simulink model "ElectricVehicleNMPC"  (R2022b)
settings: Solver=VariableStepAuto  StartTime=0  StopTime=600+N*Ts  RelTol=1e-3
model workspace (MAT data in the model file):
  AccessaryLoad : Simulink.Parameter (value not decoded)
  BrakeRegenFraction : Simulink.Parameter (value not decoded)
  Crr : Simulink.Parameter (value not decoded)
  DrivelineModelG : Simulink.Parameter (value not decoded)
  DrivelineModelSpinLoss : Simulink.Parameter (value not decoded)
  EnergyCapacity : Simulink.Parameter (value not decoded)
  MassVehInertia : Simulink.Parameter (value not decoded)
  MaxPowerOutput : Simulink.Parameter (value not decoded)
  MaxTorqueOutput : Simulink.Parameter (value not decoded)
  MaximumBreakForce : Simulink.Parameter (value not decoded)
  MotorModelC : Simulink.Parameter (value not decoded)
  MotorModelKc : Simulink.Parameter (value not decoded)
  MotorModelKi : Simulink.Parameter (value not decoded)
  MotorModelKw : Simulink.Parameter (value not decoded)
  N : Simulink.Parameter (value not decoded)
  Q : Simulink.Parameter (value not decoded)
  Rint : Simulink.Parameter (value not decoded)
  Ts : Simulink.Parameter (value not decoded)
  Voc : Simulink.Parameter (value not decoded)
  gravity : Simulink.Parameter (value not decoded)
  massVeh : Simulink.Parameter (value not decoded)
  theta : Simulink.Parameter (value not decoded)
  wheelRadius : Simulink.Parameter (value not decoded)
values from neighbouring files (symbols this model uses):
  AccessaryLoad = 600    [NMPC_EV.m]
  BrakeRegenFraction = 0.55    [NMPC_EV.m]
  Crr = 0.01    [NMPC_EV.m]
  DrivelineModelG = 3.55    [NMPC_EV.m]
  DrivelineModelSpinLoss = 6    [NMPC_EV.m]
  EnergyCapacity = 12.6    [NMPC_EV.m]
  gravity = 9.81    [NMPC_EV.m]
  m = 2    [NMPC_EV.m]
  massVeh = 2300    [NMPC_EV.m]
  MassVehInertia = 2392    [NMPC_EV.m]
  MaximumBreakForce = 10000    [NMPC_EV.m]
  MaxPowerOutput = 1e5    (= 100000)    [NMPC_EV.m]
  MaxTorqueOutput = 500    [NMPC_EV.m]
  MotorModelC = 628.2974    [NMPC_EV.m]
  MotorModelKc = 0.045237    [NMPC_EV.m]
  MotorModelKi = 0.0167    [NMPC_EV.m]
  MotorModelKw = 5.06640055940796E-5    (= 5.06640055941e-05)    [NMPC_EV.m]
  N = 5    [NMPC_EV.m]
  Q = 3000    [NMPC_EV.m]
  Rint = 0.1    [NMPC_EV.m]
  Ts = 0.01    [NMPC_EV.m]
  Voc = 340    [NMPC_EV.m]
  wheelRadius = 0.34    [NMPC_EV.m]
symbols that are objects in the model workspace (value not decoded): theta
libraries: simulink x12, autolibshared x2
(part 2 of 2)

== matlab function ElectricVehicleNMPC/NMPC1/MATLAB Function ==
  settings: updateMethod=DISCRETE
  data: Vahead input; Vref input; Pt output; FB output; VehicleV input; soc input; N data_store_memory; BrakeRegenFraction data_store_memory; Crr data_store_memory; DrivelineModelG data_store_memory; DrivelineModelSpinLoss data_store_memory; EnergyCapacity data_store_memory; MassVehInertia data_store_memory; MotorModelC data_store_memory; MotorModelKc data_store_memory; MotorModelKi data_store_memory; MotorModelKw data_store_memory; Rint data_store_memory; Voc data_store_memory; massVeh data_store_memory; wheelRadius data_store_memory; AccessaryLoad data_store_memory; Ts data_store_memory; gravity data_store_memory; Q data_store_memory; MaxTorqueOutput data_store_memory; n data_store_memory; m data_store_memory; vr data_store_memory; v data_store_memory; SOC data_store_memory; SOCr data_store_memory; Ptr data_store_memory; FBr data_store_memory; MaxPowerOutput data_store_memory; Vpre data_store_memory
function [Pt,FB] = fcn(Vahead,Vref,VehicleV,soc)
% u1 = Pt Positive Torque
% u2 = FB Total BrakeForce


global AccessaryLoad BrakeRegenFraction Crr DrivelineModelG DrivelineModelSpinLoss EnergyCapacity MassVehInertia MotorModelC
global MotorModelKc MotorModelKi MotorModelKw Rint Voc massVeh wheelRadius MaxTorqueOutput MaxPowerOutput
global N Ts Q
global n m vr v Ptr FBr SOC SOCr Vpre

persistent Vtrajectory zek G_rw u1 u2
persistent xmin xmax umin Fx Fu R Qx QX RU FX FU F H
if isempty(u1)
    G_rw = DrivelineModelG/wheelRadius;
    Vtrajectory = zeros(N+1,1); % +1 to include current reference
    zek = [zeros(n*(N+1),1);zeros(m*N,1)];

    xmin = [-1e5;5]; xmax = [1e5;100]; 
    umin = [0;-1e4];
    Fx = [0 0;0 1;0 0;0 -1]; % No constraints on velcity
    Fu = [eye(m);-eye(m)]; R = eye(m);
    Qx = [Q 0;0 1];
    QX = zeros(n*(N+1),n*(N+1));
    RU = zeros(m*N,m*N);
    FX = zeros(2*n*(N+1),n*(N+1));
    FU = zeros(2*m*N,m*N);
    for i = 1:N
        QX((i-1)*n+1:i*n,(i-1)*n+1:i*n) = Qx;
        RU((i-1)*m+1:i*m,(i-1)*m+1:i*m) = R;

        FX((i-1)*2*n+1:i*2*n,(i-1)*n+1:i*n) = Fx;
        FU((i-1)*2*m+1:i*2*m,(i-1)*m+1:i*m) = Fu;
    end
    QX(N*n+1:end,N*n+1:end) = Qx;
    FX(N*2*n+1:end,N*n+1:end) = Fx;
    F = blkdiag(FX,FU);
    H = blkdiag(QX,RU.*0); 

    SOCr=100;
    u1=0;u2=0;
end

Vtrajectory(1:end-1,1) = Vtrajectory(2:end,1);
Vtrajectory(end,1) = Vahead;
% Vpre = Vtrajectory; % from persistent variable to global variable
Vpre = zeros(11,1);
for i =1:N+1
    Vpre(i)=Vtrajectory(i,1);
end
vr = Vref; v = VehicleV; SOC = soc; 

MotorSpeed = max(G_rw*abs(v),1e-5); % MotorSpeed must be positive
umax = [min(MaxTorqueOutput,MaxPowerOutput/MotorSpeed);0];

Gxe = zeros(2*n*(N+1),1);
Gue = zeros(2*m*N,1);
Ptr=zeros(11,1);FBr=zeros(11,1);
Pt=u1;FB=u2;
for i = 1:N
    xr = [Vtrajectory(i,1);SOCr]; %future references
    [Pt,FB] = desiredControl(xr(1),Vtrajectory(i+1),Pt,FB); % Find equilibrium control using fd
    Ptr(i,1)=Pt;FBr(i,1)=FB;

    gxe = [xmax;-xmin] - Fx*xr;
    gue = [umax;-umin] - Fu*[Pt;FB];

    Gxe((i-1)*2*n+1:i*2*n,1) = gxe;
    Gue((i-1)*2*m+1:i*2*m,1) = gue;
end
xr = [Vtrajectory(end,1);SOCr]; %future references
[Ptr(end,1),FBr(end,1)] = desiredControl(xr(1),xr(1),Pt,FB);
gxe = [xmax;-xmin] - Fx*xr;
Gxe(N*2*n+1:end,1) = gxe;

% Simulation with NMPC
ObjFunc = @(ze) (ze'*H*ze);
G = [Gxe;Gue];
nonlcon = @NonlinearConstraints;
options = optimoptions('fmincon','Algorithm','sqp');
zek = fmincon(ObjFunc,zek,F,G,[],[],[],[],nonlcon,options);
u = zek(n*(N+1)+1:n*(N+1)+m,1) + [Ptr(1,1);FBr(1,1)];
% if(abs(vr)==abs(v))
%     u1=0;u2=0;
% elseif(vr>v)
%     u1=u(1);
%     u2=0;
% else
%     u1=0;
%     u2=u(2);
% end
if(abs(vr)==abs(v)&&abs(v)==0)
    u1=0;u2=0;
else
    u1=u(1);u2=u(2);
end
Pt = u1;
FB = u2;
end


%%%%%%%%%%%%%%%%%%%%%%%%%%%%%%%%%%%%%%%%%%%%%%%%%%%%%%%%%%%%%%%%%%%%%%%%%%%
%%%%%%%%%%%%%%%%%%%%%%%%%%%%%%%%%%%%%%%%%%%%%%%%%%%%%%%%%%%%%%%%%%%%%%%%%%%
function [Ptr, FBr] = desiredControl(vr,vr1,Pt,FB)
global massVeh gravity Crr DrivelineModelSpinLoss DrivelineModelG wheelRadius MassVehInertia
global BrakeRegenFraction AccessaryLoad  MotorModelKc MotorModelKw MotorModelKi MotorModelC Ts

G_rw = DrivelineModelG/wheelRadius;
C1 = 0.5*vr^2 + massVeh*gravity*Crr + DrivelineModelSpinLoss*G_rw;
C2 = AccessaryLoad + MotorModelKw*(G_rw*vr)^3 + MotorModelKi*G_rw*vr + MotorModelC;
root = roots([MotorModelKc,G_rw*vr,C2]);
if(isreal(root))
    TM_r = max(root);
    u2r = C1 - TM_r*G_rw + (vr1-vr)*MassVehInertia/Ts;
    u1r = TM_r + BrakeRegenFraction/G_rw*u2r;

%     Ptr = max(0,u1r);
%     FBr = min(0,u2r);
    Ptr = u1r;
    FBr = u2r;
else
    Ptr = Pt;
    FBr = FB;
end

end

function [c,ceq] = NonlinearConstraints(z)
global v SOC SOCr Ptr FBr Vpre
global N n m
c=[];
shift = n*(N+1);
c1 = zeros(n*N,1);
for i=1:N
    vz = z(n*(i-1)+1,1);
    socz = z(i*n,1);
    Ptz = z(shift+m*(i-1)+1,1);
    FBz = z(shift+i*m,1);
    Pt_r = Ptr(i);FB_r=FBr(i);v_r=Vpre(i,1);
    [v1,soc1] = fd2(vz+v_r,socz+SOCr,Ptz+Pt_r,FBz+FB_r);
    c1(n*(i-1)+1) = z(i*n+1,1)+v_r - v1;
    c1(n*i) = z((i+1)*n,1)+SOCr - soc1;
end
ceq = [z(1)+Vpre(1,1)-v;z(2)+SOCr-SOC;c1];
end

function [v_prime,soc_prime] = fd2(v,SOC,PositiveTorque,FB)
global Ts
[dv1,dsoc1] = fc(v,PositiveTorque,FB);
v_prime = v + Ts*dv1;
soc_prime = SOC + Ts*dsoc1;
end

function [dv,dsoc] = fc(v,PositiveTorque,FB)
global MassVehInertia massVeh gravity Crr DrivelineModelSpinLoss DrivelineModelG
global wheelRadius BrakeRegenFraction Voc EnergyCapacity MaxTorqueOutput MaxPowerOutput

G_wr = DrivelineModelG/wheelRadius;
MotorSpeed = max(G_wr*abs(v),1e-5);
if(abs(v)<2.2352) % less than 2.2352 m/s = 5mph
    RegenTorque = 0;
else
    RegenTorque = BrakeRegenFraction*FB/G_wr; % Negative
    RegenTorque = max(RegenTorque,-0.5*min(MaxTorqueOutput,MaxPowerOutput/MotorSpeed));
end
BrakeForce = max((1-BrakeRegenFraction)*FB,-1e4);
MotorTorque = PositiveTorque + RegenTorque;
if(abs(v)~=0)
    TractiveForce = (MotorTorque - DrivelineModelSpinLoss)*G_wr  + BrakeForce;
    RollingResistence = massVeh*gravity*Crr;
else
    TractiveForce = MotorTorque*G_wr  + BrakeForce;
    RollingResistence = 0;
end
dv = (TractiveForce - 0.5*v^2 -RollingResistence)/MassVehInertia;
P = MotorPower(MotorTorque,MotorSpeed);
I = Current(P);
dsoc = -Voc*I/(EnergyCapacity*1000*3600)*100;% in %
end

function P = MotorPower(MotorTorque,MotorSpeed)
global AccessaryLoad  MotorModelKc MotorModelKw MotorModelKi MotorModelC 
if(MotorSpeed>1e-3)
    Powerloss = MotorModelKc*MotorTorque^2 +... 
         MotorModelKw*(MotorSpeed)^3 + MotorModelKi*MotorSpeed + MotorModelC;
else
    Powerloss =  0;
end
P = Powerloss + MotorSpeed*MotorTorque + AccessaryLoad;
end

function I = Current(P)
global Voc Rint
dummy = Voc^2 - 4*Rint*P;
I = (Voc - sqrt(dummy))/(2*Rint);
end

== matlab function ElectricVehicleNMPC/NMPC/MATLAB Function ==
  settings: updateMethod=DISCRETE
  data: Vahead input; Vref input; Pt output; FB output; VehicleV input; soc input; N data_store_memory; BrakeRegenFraction data_store_memory; Crr data_store_memory; DrivelineModelG data_store_memory; DrivelineModelSpinLoss data_store_memory; EnergyCapacity data_store_memory; MassVehInertia data_store_memory; MotorModelC data_store_memory; MotorModelKc data_store_memory; MotorModelKi data_store_memory; MotorModelKw data_store_memory; Rint data_store_memory; Voc data_store_memory; massVeh data_store_memory; wheelRadius data_store_memory; AccessaryLoad data_store_memory; Ts data_store_memory; gravity data_store_memory; Q data_store_memory; MaxTorqueOutput data_store_memory; n data_store_memory; m data_store_memory; vr data_store_memory; v data_store_memory; SOC data_store_memory; SOCr data_store_memory; Ptr data_store_memory; FBr data_store_memory; MaxPowerOutput data_store_memory; Vpre data_store_memory
function [Pt,FB] = fcn(Vahead,Vref,VehicleV,soc)
% u1 = Pt Positive Torque
% u2 = FB Total BrakeForce


global AccessaryLoad BrakeRegenFraction Crr DrivelineModelG DrivelineModelSpinLoss EnergyCapacity MassVehInertia MotorModelC
global MotorModelKc MotorModelKi MotorModelKw Rint Voc massVeh wheelRadius MaxTorqueOutput MaxPowerOutput
global N Ts Q
global n m vr v Ptr FBr SOC SOCr Vpre

persistent Vtrajectory zek G_rw u1 u2
persistent xmin xmax umin Fx Fu R Qx QX RU FX FU F H
if isempty(u1)
    G_rw = DrivelineModelG/wheelRadius;
    Vtrajectory = zeros(N+1,1); % +1 to include current reference
    zek = [zeros(n*(N+1),1);zeros(m*N,1)];

    xmin = [-1e5;5]; xmax = [1e5;100]; 
    umin = [0;-1e4];
    Fx = [0 0;0 1;0 0;0 -1]; % No constraints on velcity
    Fu = [eye(m);-eye(m)]; R = eye(m);
    Qx = [Q 0;0 1];
    QX = zeros(n*(N+1),n*(N+1));
    RU = zeros(m*N,m*N);
    FX = zeros(2*n*(N+1),n*(N+1));
    FU = zeros(2*m*N,m*N);
    for i = 1:N
        QX((i-1)*n+1:i*n,(i-1)*n+1:i*n) = Qx;
        RU((i-1)*m+1:i*m,(i-1)*m+1:i*m) = R;

        FX((i-1)*2*n+1:i*2*n,(i-1)*n+1:i*n) = Fx;
        FU((i-1)*2*m+1:i*2*m,(i-1)*m+1:i*m) = Fu;
    end
    QX(N*n+1:end,N*n+1:end) = Qx;
    FX(N*2*n+1:end,N*n+1:end) = Fx;
    F = blkdiag(FX,FU);
    H = blkdiag(QX,RU.*0); 

    SOCr=100;
    u1=0;u2=0;
end

Vtrajectory(1:end-1,1) = Vtrajectory(2:end,1);
Vtrajectory(end,1) = Vahead;
% Vpre = Vtrajectory; % from persistent variable to global variable
Vpre = zeros(11,1);
for i =1:N+1
    Vpre(i)=Vtrajectory(i,1);
end
vr = Vref; v = VehicleV; SOC = soc; 

MotorSpeed = max(G_rw*abs(v),1e-5); % MotorSpeed must be positive
umax = [min(MaxTorqueOutput,MaxPowerOutput/MotorSpeed);0];

Gxe = zeros(2*n*(N+1),1);
Gue = zeros(2*m*N,1);
Ptr=zeros(11,1);FBr=zeros(11,1);
Pt=u1;FB=u2;
for i = 1:N
    xr = [Vtrajectory(i,1);SOCr]; %future references
    [Pt,FB] = desiredControl(xr(1),Vtrajectory(i+1),Pt,FB); % Find equilibrium control using fd
    Ptr(i,1)=Pt;FBr(i,1)=FB;

    gxe = [xmax;-xmin] - Fx*xr;
    gue = [umax;-umin] - Fu*[Pt;FB];

    Gxe((i-1)*2*n+1:i*2*n,1) = gxe;
    Gue((i-1)*2*m+1:i*2*m,1) = gue;
end
xr = [Vtrajectory(end,1);SOCr]; %future references
[Ptr(end,1),FBr(end,1)] = desiredControl(xr(1),xr(1),Pt,FB);
gxe = [xmax;-xmin] - Fx*xr;
Gxe(N*2*n+1:end,1) = gxe;

% Simulation with NMPC
ObjFunc = @(ze) (ze'*H*ze);
G = [Gxe;Gue];
nonlcon = @NonlinearConstraints;
options = optimoptions('fmincon','Algorithm','sqp');
zek = fmincon(ObjFunc,zek,F,G,[],[],[],[],nonlcon,options);
u = zek(n*(N+1)+1:n*(N+1)+m,1) + [Ptr(1,1);FBr(1,1)];
% if(abs(vr)==abs(v))
%     u1=0;u2=0;
% elseif(vr>v)
%     u1=u(1);
%     u2=0;
% else
%     u1=0;
%     u2=u(2);
% end
if(abs(vr)==abs(v)&&abs(v)==0)
    u1=0;u2=0;
else
    u1=u(1);u2=u(2);
end
Pt = u1;
FB = u2;
end


%%%%%%%%%%%%%%%%%%%%%%%%%%%%%%%%%%%%%%%%%%%%%%%%%%%%%%%%%%%%%%%%%%%%%%%%%%%
%%%%%%%%%%%%%%%%%%%%%%%%%%%%%%%%%%%%%%%%%%%%%%%%%%%%%%%%%%%%%%%%%%%%%%%%%%%
function [Ptr, FBr] = desiredControl(vr,vr1,Pt,FB)
global massVeh gravity Crr DrivelineModelSpinLoss DrivelineModelG wheelRadius MassVehInertia
global BrakeRegenFraction AccessaryLoad  MotorModelKc MotorModelKw MotorModelKi MotorModelC Ts

G_rw = DrivelineModelG/wheelRadius;
C1 = 0.5*vr^2 + massVeh*gravity*Crr + DrivelineModelSpinLoss*G_rw;
C2 = AccessaryLoad + MotorModelKw*(G_rw*vr)^3 + MotorModelKi*G_rw*vr + MotorModelC;
root = roots([MotorModelKc,G_rw*vr,C2]);
if(isreal(root))
    TM_r = max(root);
    u2r = C1 - TM_r*G_rw + (vr1-vr)*MassVehInertia/Ts;
    u1r = TM_r + BrakeRegenFraction/G_rw*u2r;

%     Ptr = max(0,u1r);
%     FBr = min(0,u2r);
    Ptr = u1r;
    FBr = u2r;
else
    Ptr = Pt;
    FBr = FB;
end

end

function [c,ceq] = NonlinearConstraints(z)
global v SOC SOCr Ptr FBr Vpre
global N n m
c=[];
shift = n*(N+1);
c1 = zeros(n*N,1);
for i=1:N
    vz = z(n*(i-1)+1,1);
    socz = z(i*n,1);
    Ptz = z(shift+m*(i-1)+1,1);
    FBz = z(shift+i*m,1);
    Pt_r = Ptr(i);FB_r=FBr(i);v_r=Vpre(i,1);
    [v1,soc1] = fd2(vz+v_r,socz+SOCr,Ptz+Pt_r,FBz+FB_r);
    c1(n*(i-1)+1) = z(i*n+1,1)+v_r - v1;
    c1(n*i) = z((i+1)*n,1)+SOCr - soc1;
end
ceq = [z(1)+Vpre(1,1)-v;z(2)+SOCr-SOC;c1];
end

function [v_prime,soc_prime] = fd2(v,SOC,PositiveTorque,FB)
global Ts
[dv1,dsoc1] = fc(v,PositiveTorque,FB);
v_prime = v + Ts*dv1;
soc_prime = SOC + Ts*dsoc1;
end

function [dv,dsoc] = fc(v,PositiveTorque,FB)
global MassVehInertia massVeh gravity Crr DrivelineModelSpinLoss DrivelineModelG
global wheelRadius BrakeRegenFraction Voc EnergyCapacity MaxTorqueOutput MaxPowerOutput

G_wr = DrivelineModelG/wheelRadius;
MotorSpeed = max(G_wr*abs(v),1e-5);
if(abs(v)<2.2352) % less than 2.2352 m/s = 5mph
    RegenTorque = 0;
else
    RegenTorque = BrakeRegenFraction*FB/G_wr; % Negative
    RegenTorque = max(RegenTorque,-0.5*min(MaxTorqueOutput,MaxPowerOutput/MotorSpeed));
end
BrakeForce = max((1-BrakeRegenFraction)*FB,-1e4);
MotorTorque = PositiveTorque + RegenTorque;
if(abs(v)~=0)
    TractiveForce = (MotorTorque - DrivelineModelSpinLoss)*G_wr  + BrakeForce;
    RollingResistence = massVeh*gravity*Crr;
else
    TractiveForce = MotorTorque*G_wr  + BrakeForce;
    RollingResistence = 0;
end
dv = (TractiveForce - 0.5*v^2 -RollingResistence)/MassVehInertia;
P = MotorPower(MotorTorque,MotorSpeed);
I = Current(P);
dsoc = -Voc*I/(EnergyCapacity*1000*3600)*100;% in %
end

function P = MotorPower(MotorTorque,MotorSpeed)
global AccessaryLoad  MotorModelKc MotorModelKw MotorModelKi MotorModelC 
if(MotorSpeed>1e-3)
    Powerloss = MotorModelKc*MotorTorque^2 +... 
         MotorModelKw*(MotorSpeed)^3 + MotorModelKi*MotorSpeed + MotorModelC;
else
    Powerloss =  0;
end
P = Powerloss + MotorSpeed*MotorTorque + AccessaryLoad;
% if(P>1e4)
%     [MotorTorque MotorSpeed]
% end
end

function I = Current(P)
global Voc Rint
dummy = Voc^2 - 4*Rint*P;
I = (Voc - sqrt(dummy))/(2*Rint);
end
